simulink model "Tema1"  (R2023b)
settings: Solver=VariableStepAuto  StartTime=0.0  StopTime=1000  RelTol=1e-3
values from neighbouring files (symbols this model uses):
  a1 = 4.2175 * 10^(-5)    (= 4.2175e-05)    [Script_Tema_1_MS.m]
  A2 = 0.021    [Script_Tema_1_MS.m]
  a2 = 4.4842 * 10^(-5)    (= 4.4842e-05)    [Script_Tema_1_MS.m]
  ac = 4.307 * 10^(-6)    (= 4.307e-06)    [Script_Tema_1_MS.m]
  AT = 0.1273    [Script_Tema_1_MS.m]
  g = 9.8    [Script_Tema_1_MS.m]
  H = 0.25    [Script_Tema_1_MS.m]
  l = 0.14    [Script_Tema_1_MS.m]
  L = 0.08    [Script_Tema_1_MS.m]
  Qin1 = Qs    [Script_Tema_1_MS.m]
  Qin2 = Qd    [Script_Tema_1_MS.m]
  Qp1 = 0.5 * 10^(-4)    (= 5e-05)    [Script_Tema_1_MS.m]
  Qp2 = 0.5 * 10^(-4)    (= 5e-05)    [Script_Tema_1_MS.m]
  teta = pi/12    (= 0.261799387799)    [Script_Tema_1_MS.m]
settings Model: Creator=bogda  LastModifiedBy=Alex

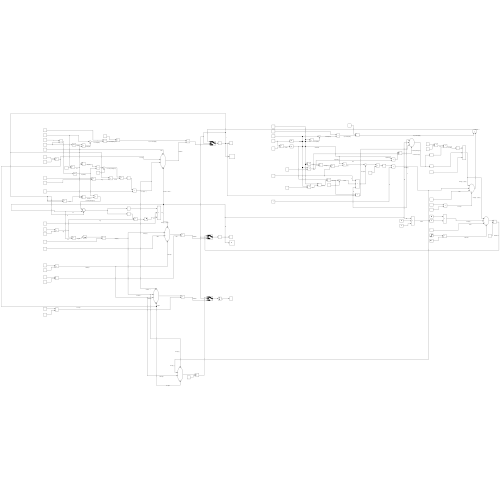
[thumbnail: Simulink's stored preview of the top-level diagram]
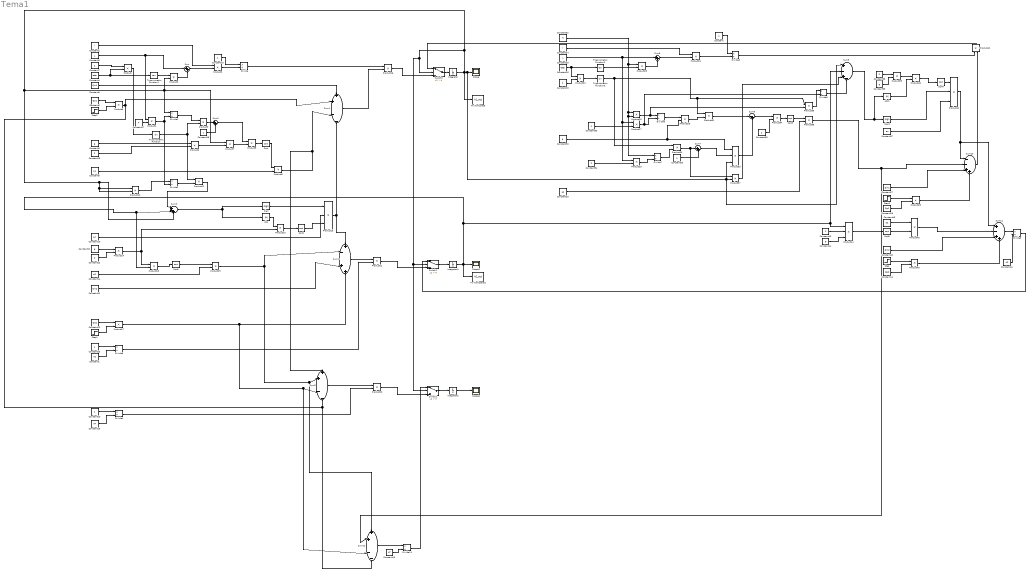
== system Tema1 ==
  Abs : Abs  SaturateOnIntegerOverflow=off
  Abs1 : Abs  SaturateOnIntegerOverflow=off
  Constant{,16,18,20,23,35} (6 alike) : Constant
  Constant1 : Constant  Value=A2
  Constant10 : Constant  Value=ac
  Constant11 : Constant  Value=Qin2
  Constant12 : Constant  Value=Qp2
  Constant{7,13,19,22,34,36,38,43} (8 alike) : Constant  Value=2
  Constant14 : Constant  Value=a2
  Constant15 : Constant  Value=AT
  Constant17 : Constant  Value=4
  Constant2 : Constant  Value=l
  Constant{9,21,30,39,44} (5 alike) : Constant  Value=g
  Constant24 : Constant  Value=l
  Constant25 : Constant  Value=L
  Constant26 : Constant  Value=teta
  Constant27 : Constant  Value=Qin1
  Constant28 : Constant  Value=Qp1
  Constant29 : Constant  Value=a1
  Constant3 : Constant  Value=L
  Constant32 : Constant  Value=H
  Constant33 : Constant  Value=4
  Constant37 : Constant  Value=ac
  Constant4 : Constant  Value=teta
  Constant40 : Constant  Value=Qin2
  Constant41 : Constant  Value=Qp2
  Constant45 : Constant  Value=a2
  Constant46 : Constant  Value=A2
  Constant49 : Constant  Value=AT
  Constant5 : Constant  Value=Qin1
  Constant6 : Constant  Value=Qp1
  Constant8 : Constant  Value=a1
  Divide{,1..9,11} (11 alike) : Product  Inputs=*/
  Integrator : Integrator  InitialCondition=0.1
  Integrator1 : Integrator
  Integrator2 : Integrator  InitialCondition=1
  Product{,1..11,13..14,16..31,34..37,39..40,42..43,45} (39 alike) : Product
  Product{15,33,41,44} (4 alike) : Product  Inputs=3
  Scope : Scope
  Scope1 : Scope
  Scope2 : Scope
  Sign : Signum
  Sign1 : Signum
  Sqrt{,1..5} (6 alike) : Sqrt
  Step{,1..3} (4 alike) : Step  After=5  SampleTime=0
  Sum{,2,6..7} (4 alike) : Sum  Inputs=|++
  Sum1 : Sum  Inputs=++--
  Sum10 : Sum  Inputs=|--++
  Sum11 : Sum  Inputs=|+-++
  Sum12 : Sum  Inputs=++--
  Sum3 : Sum  Inputs=|+-+
  Sum4 : Sum  Inputs=+-++
  Sum5 : Sum  Inputs=++--
  Sum8 : Sum  Inputs=|-+
  Sum9 : Sum  Inputs=|+-+-
  Switch1 : Switch  Criteria=u2 > Threshold  Threshold=H  SaturateOnIntegerOverflow=off  InputSameDT=off
  Switch2 : Switch  Criteria=u2 > Threshold  Threshold=H  SaturateOnIntegerOverflow=off  InputSameDT=off
  Switch3 : Switch  Criteria=u2 > Threshold  Threshold=H  SaturateOnIntegerOverflow=off  InputSameDT=off
  To Workspace : ToWorkspace  VariableName=h1_out  SampleTime=-1
      settings: Save2DSignal=2-D array (concatenate along first dimension)
  To Workspace1 : ToWorkspace  VariableName=h2_out  SampleTime=-1
      settings: Save2DSignal=2-D array (concatenate along first dimension)
  Trigonometric Function : Trigonometry
  Trigonometric Function1 : Trigonometry  Operator=tan
  Trigonometric Function2 : Trigonometry  Operator=tan
  Trigonometric Function3 : Trigonometry
  wires:
  Constant4/1 -> Product/2, Trigonometric Function1/1
  Product/1 -> Trigonometric Function/1
  Integrator/1 -> To Workspace/1, Product33/3, Sum9/1, Product37/2, Scope/1, Product7/1, Product1/2, Divide1/1, Sum3/3, Product10/1, Product10/2, Switch3/2, Switch2/2, Switch1/2  "h1"
  Trigonometric Function1/1 -> Product1/1  "tan(teta)"
  Constant3/1 -> Product4/1, Sum/1  "L"
  Product1/1 -> Sum/2  "h1*tan(teta)"
  Sum/1 -> Product2/2  "L+h1*tan(teta)"
  Constant2/1 -> Product2/1  "l"
  Constant16/1 -> Divide/1
  Product2/1 -> Divide/2  "l*(L+h1*tan(teta))"
  Constant5/1 -> Sum1/1  "Qin1"
  Constant6/1 -> Product3/1
  Step2/1 -> Product3/2
  Constant17/1 -> Product4/2
  Product4/1 -> Divide2/2, Divide1/2  "4*L"
  Divide1/1 -> Product5/1  "h1/(4*L)"
  Trigonometric Function/1 -> Product5/2, Product11/1  "sin(2*teta)"
  Product5/1 -> Sum2/1
  Constant18/1 -> Sum2/2
  Constant9/1 -> Product6/1
  Constant19/1 -> Product6/2
  Product6/1 -> Product7/2  "2*g"
  Product7/1 -> Product8/2  "2*g*h1"
  Sum2/1 -> Product8/1  "1+ h1*sin(2*teta)/(4*L)"
  Product8/1 -> Sqrt/1
  Constant8/1 -> Product9/2
  Sqrt/1 -> Product9/1
  Product9/1 -> Sum5/1, Sum1/3  "a1*sqrt(....)"
  Product10/1 -> Divide2/1  "h1^2"
  Divide2/1 -> Product11/2  "h1^2/(4*L)"
  Product11/1 -> Sum3/1  "h1^2*sin(2*teta)/(4*L)"
  Sum3/1 -> Abs/1, Sign/1
  Sign/1 -> Product15/1
  Constant10/1 -> Product15/2  "ac"
  Constant21/1 -> Product14/1
  Constant22/1 -> Product14/2
  Product14/1 -> Product18/1, Product13/2  "2*g"
  Abs/1 -> Product13/1
  Product13/1 -> Sqrt1/1
  Product15/1 -> Sum4/1, Sum1/4  "ac*sign(...)*sqrt(...)"
  Divide/1 -> Product16/1  "1/l*(L+h1*tan(teta))"
  Sum1/1 -> Product16/2  "Relatia1"
  Product16/1 -> Switch3/3
  Switch3/1 -> Integrator/1
  Constant23/1 -> Divide3/1
  Constant1/1 -> Divide3/2
  Constant12/1 -> Product17/1
  Step1/1 -> Product17/2
  Constant11/1 -> Sum4/3  "Qin2"
  Product18/1 -> Sqrt2/1  "2*g*h2"
  Constant14/1 -> Product19/2
  Sqrt2/1 -> Product19/1
  Product17/1 -> Sum12/3, Sum5/3, Sum4/4  "u22*Qp2"
  Divide3/1 -> Product21/2  "1/A2"
  Sum4/1 -> Product21/1
  Product21/1 -> Switch1/3  "Relatia2"
  Switch1/1 -> Integrator1/1
  Integrator1/1 -> To Workspace1/1, Product44/1, Sum9/2, Product18/2, Sum3/2, Scope1/1  "h2"
  Product3/1 -> Sum5/4, Sum12/4, Sum1/2  "u11*Qp1"
  Constant20/1 -> Divide4/1
  Constant15/1 -> Divide4/2
  Sum5/1 -> Product20/1
  Divide4/1 -> Product20/2
  Product20/1 -> Switch2/3  "Relatia3"
  Switch2/1 -> Integrator2/1
  Integrator2/1 -> Scope2/1  "h"
  Product22/1 -> Trigonometric Function3/1  "2*teta"
  Constant26/1 -> Trigonometric Function2/1, Product22/1
  Trigonometric Function2/1 -> Product23/2  "tan(teta)"
  Constant32/1 -> Divide7/1, Product26/2, Product26/1, Product23/1  "H"
  Constant25/1 -> Product29/1, Product27/1, Sum6/1
  Product23/1 -> Sum6/2  "H*tan(teta)"
  Sum6/1 -> Product24/2  "L+H*tan(teta)"
  Constant24/1 -> Product24/1
  Product24/1 -> Divide5/2  "l*(L+H*tan(teta))"
  Constant/1 -> Divide5/1
  Step3/1 -> Product25/1
  Constant28/1 -> Product25/2
  Constant33/1 -> Product27/2
  Product26/1 -> Product36/2, Divide6/1  "H^2"
  Product27/1 -> Divide8/2, Divide6/2  "4*L"
  Divide6/1 -> Product28/1  "H^2/(4*L)"
  Constant30/1 -> Product33/1, Product28/2  "g"
  Constant34/1 -> Product29/2
  Product29/1 -> Divide7/2  "2*L"
  Trigonometric Function3/1 -> Product31/1, Product36/1, Product30/1  "sin(2*teta)"
  Product28/1 -> Product31/2
  Product31/1 -> Sum8/1  "g*(...)"
  Divide7/1 -> Product30/2  "H/(2*L)"
  Product30/1 -> Product37/1, Sum7/1  "H/2L*sin"
  Constant35/1 -> Sum7/2
  Sum7/1 -> Product33/2  "1+ceva"
  Product33/1 -> Sum8/2
  Sum8/1 -> Product34/1
  Constant36/1 -> Product34/2
  Product34/1 -> Sqrt3/1
  Sqrt3/1 -> Product35/1
  Constant29/1 -> Product35/2  "a1"
  Product36/1 -> Divide8/1
  Divide8/1 -> Sum9/4  "H^2*sin(2*teta)/(4*L)"
  Product37/1 -> Sum9/3  "h1*H/(2*L)"
  Sum9/1 -> Abs1/1, Sign1/1  "ce se afla in sign"
  Sign1/1 -> Product41/2
  Constant37/1 -> Product41/3
  Constant38/1 -> Product39/1
  Constant39/1 -> Product39/2
  Product39/1 -> Product40/1  "2*g"
  Abs1/1 -> Product40/2
  Product40/1 -> Sqrt4/1  "2*g*abs"
  Sqrt4/1 -> Product41/1
  Product35/1 -> Sum12/2, Sum10/2  "a1*sqrt(...)"
  Constant27/1 -> Sum10/3  "Qin1"
  Product25/1 -> Sum10/4  "u11*Qp1"
  Sum10/1 -> Product42/2
  Divide5/1 -> Product42/1  "1/l*(L+H*tan(teta))"
  Product42/1 -> Switch3/1  "Relatia1.1"
  Product41/1 -> Sum11/1, Sum10/1  "ac*sign(...)*sqrt(...)"
  Step/1 -> Product43/1
  Constant41/1 -> Product43/2
  Product43/1 -> Sum11/4  "Qp2*u22"
  Constant40/1 -> Sum11/3  "Qin2"
  Constant43/1 -> Product44/2
  Constant44/1 -> Product44/3
  Product44/1 -> Sqrt5/1  "2*g*h2"
  Constant45/1 -> Product45/1
  Sqrt5/1 -> Product45/2
  Product45/1 -> Sum11/2  "a2*sqrt(...)"
  Sum11/1 -> Divide9/1
  Constant46/1 -> Divide9/2
  Divide9/1 -> Switch1/1  "Relatia2.2"
  Product19/1 -> Sum5/2, Sum12/1, Sum4/2  "a2*sqrt(...)"
  Sum12/1 -> Divide11/1
  Constant49/1 -> Divide11/2
  Divide11/1 -> Switch2/1
  Constant7/1 -> Product/1
  Constant13/1 -> Product22/2
  Sqrt1/1 -> Product15/3
